simulink model "Receiver_model"  (R2021b)
settings: Solver=FixedStepAuto  StartTime=0  StopTime=70670*4  FixedStep=1  RelTol=1e-3
PostLoadFcn:
  | VarLoad
InitFcn:
  | VarLoad
model workspace: external: MAT-File D:\NIR\WIFI\AGC\Simulink_model\ex1.mat (data not in the file)
undefined symbols (not defined in the file or in its folder): F, magnitude, STF
libraries: simulink x4, dspmathops x1, hdlsllib x1
settings Model: SimulationMode=accelerator  Creator=vadim  LastModifiedBy=vadim

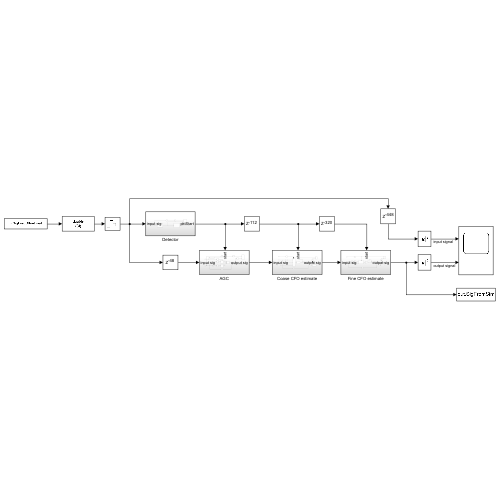
[thumbnail: Simulink's stored preview of the top-level diagram]
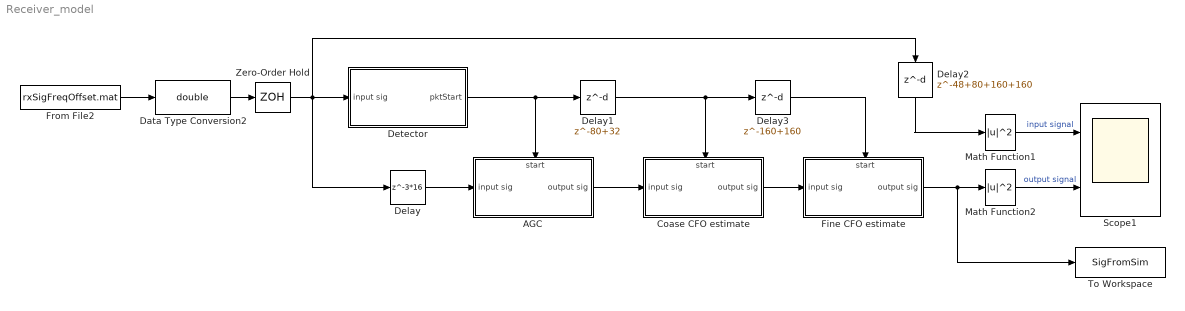
== system Receiver_model ==
  AGC : Subsystem
      settings: PortSchema="{\"entries\":[{\"content\":{\"sides\":[{\"content\":{\"connectorIds\":[\"In1\"]},\"type\":\"ConnectorPlacement.EquallySpacedRectSide\",\"uuid\":\"8c7787f9-30c4-4d5b-a9f2-4534fe769227\"},{\"content\":{\"connectorIds\":[\"Out1\"],\"side\":\"RIGHT\"},\"type\":\"ConnectorPlacement.EquallySpacedRectSide\",\"uuid\":\"2fc322a7-640d-4810-b499-987bf1f99166\"},{\"content\":{\"connectorIds\":[\"In2\"],\"side\":\"TOP\"},\"type\":\"ConnectorPlacement.EquallySpacedRectSide\",\"uuid\":\"709cb384-5402-4f06-933f-6325852d1b42\"}]},\"type\":\"ConnectorPlacement.EquallySpacedConnector\",\"uuid\":\"5f513f7d-d5a1-4295-af52-6e74ab8560d1\"}],\"packageUris\":[\"http://schema.mathworks.com/mf0/Connector/R2020b\"],\"version\":\"1.0\"}"
  Coase CFO estimate : Subsystem
      settings: PortSchema="{\"entries\":[{\"content\":{\"sides\":[{\"content\":{\"connectorIds\":[\"In1\"]},\"type\":\"ConnectorPlacement.EquallySpacedRectSide\",\"uuid\":\"8c7787f9-30c4-4d5b-a9f2-4534fe769227\"},{\"content\":{\"connectorIds\":[\"Out1\"],\"side\":\"RIGHT\"},\"type\":\"ConnectorPlacement.EquallySpacedRectSide\",\"uuid\":\"2fc322a7-640d-4810-b499-987bf1f99166\"},{\"content\":{\"connectorIds\":[\"In2\"],\"side\":\"TOP\"},\"type\":\"ConnectorPlacement.EquallySpacedRectSide\",\"uuid\":\"709cb384-5402-4f06-933f-6325852d1b42\"}]},\"type\":\"ConnectorPlacement.EquallySpacedConnector\",\"uuid\":\"5f513f7d-d5a1-4295-af52-6e74ab8560d1\"}],\"packageUris\":[\"http://schema.mathworks.com/mf0/Connector/R2020b\"],\"version\":\"1.0\"}"
  Data Type Conversion2 : DataTypeConversion  OutDataTypeStr=double  ConvertRealWorld=Stored Integer (SI)
  Delay : Delay  DelayLength=3*16
  Delay1 : Delay  DelayLength=80+32
  Delay2 : Delay  DelayLength=48+80+160+160
  Delay3 : Delay  DelayLength=160+160
  Detector : Subsystem
  Fine CFO estimate : Subsystem
      settings: PortSchema="{\"entries\":[{\"content\":{\"sides\":[{\"content\":{\"connectorIds\":[\"In1\"]},\"type\":\"ConnectorPlacement.EquallySpacedRectSide\",\"uuid\":\"8c7787f9-30c4-4d5b-a9f2-4534fe769227\"},{\"content\":{\"connectorIds\":[\"Out1\"],\"side\":\"RIGHT\"},\"type\":\"ConnectorPlacement.EquallySpacedRectSide\",\"uuid\":\"2fc322a7-640d-4810-b499-987bf1f99166\"},{\"content\":{\"connectorIds\":[\"In2\"],\"side\":\"TOP\"},\"type\":\"ConnectorPlacement.EquallySpacedRectSide\",\"uuid\":\"709cb384-5402-4f06-933f-6325852d1b42\"}]},\"type\":\"ConnectorPlacement.EquallySpacedConnector\",\"uuid\":\"5f513f7d-d5a1-4295-af52-6e74ab8560d1\"}],\"packageUris\":[\"http://schema.mathworks.com/mf0/Connector/R2020b\"],\"version\":\"1.0\"}"
  From File2 : FromFile  FileName=rxSigFreqOffset.mat  SampleTime=0  ExtrapolationAfterLastDataPoint=Ground value
  Math Function1 : Math  Operator=magnitude^2  SaturateOnIntegerOverflow=on
  Math Function2 : Math  Operator=magnitude^2  SaturateOnIntegerOverflow=on
  Scope1 : Scope  NumInputPorts=2
  To Workspace : ToWorkspace  VariableName=SigFromSim  SaveFormat=Timeseries  SampleTime=-1
  Zero-Order Hold : ZeroOrderHold
  wires:
  From File2/1 -> Data Type Conversion2/1
  Data Type Conversion2/1 -> Zero-Order Hold/1
  Delay/1 -> AGC/1(input sig)
  Zero-Order Hold/1 -> Delay/1, Delay2/1, Detector/1(input sig)
  Math Function2/1 -> Scope1/2  "output signal"
  Math Function1/1 -> Scope1/1  "input signal"
  Delay2/1 -> Math Function1/1
  AGC/1(output sig) -> Coase CFO estimate/1(input sig)
  Delay1/1 -> Delay3/1, Coase CFO estimate/2(start)
  Detector/1(pktStart) -> AGC/2(start), Delay1/1
  Coase CFO estimate/1(output sig) -> Fine CFO estimate/1(input sig)
  Fine CFO estimate/1(output sig) -> To Workspace/1, Math Function2/1
  Delay3/1 -> Fine CFO estimate/2(start)

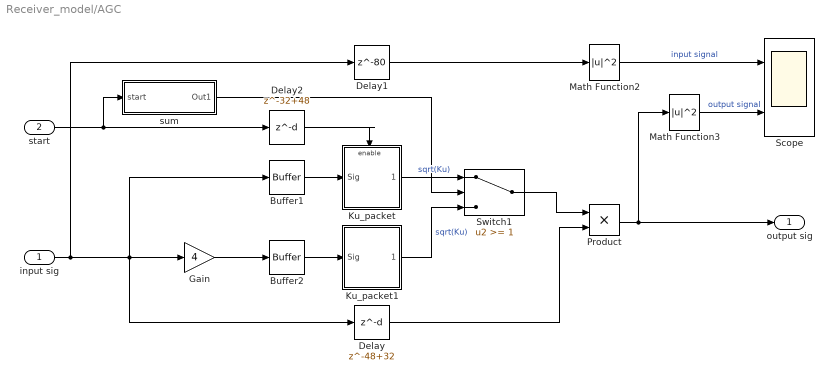
== system Receiver_model/AGC ==
  input sig : Inport
  start : Inport  Port=2
  Buffer1 : Buffer  N=3*16  V=3*16-1  OutputFrames=off
  Buffer2 : Buffer  N=3*16  V=3*16-1  OutputFrames=off
  Delay : Delay  DelayLength=48+32
  Delay1 : Delay  DelayLength=80
  Delay2 : Delay  DelayLength=32+48
  Gain : Gain  Gain=4
  Ku_packet : Subsystem
  Ku_packet1 : Subsystem
  Math Function2 : Math  Operator=magnitude^2  SaturateOnIntegerOverflow=on
  Math Function3 : Math  Operator=magnitude^2  SaturateOnIntegerOverflow=on
  Product : Product
  Scope : Scope  NumInputPorts=2
  Switch1 : Switch  Threshold=1
  sum : Subsystem
  output sig : Outport
  wires:
  Product/1 -> Math Function3/1, output sig/1
  Math Function2/1 -> Scope/1  "input signal"
  Math Function3/1 -> Scope/2  "output signal"
  Ku_packet/1(sqrt(Ku)) -> Switch1/1  "sqrt(Ku)"
  Delay/1 -> Product/2
  Delay1/1 -> Math Function2/1
  Buffer1/1 -> Ku_packet/1(Sig)
  Gain/1 -> Buffer2/1
  input sig/1 -> Delay1/1, Buffer1/1, Delay/1, Gain/1
  Delay2/1 -> Ku_packet/Enable
  Switch1/1 -> Product/1
  Buffer2/1 -> Ku_packet1/1(Sig)
  Ku_packet1/1(sqrt(Ku)) -> Switch1/3  "sqrt(Ku)"
  start/1 -> sum/1(start), Delay2/1
  sum/1(Out1) -> Switch1/2

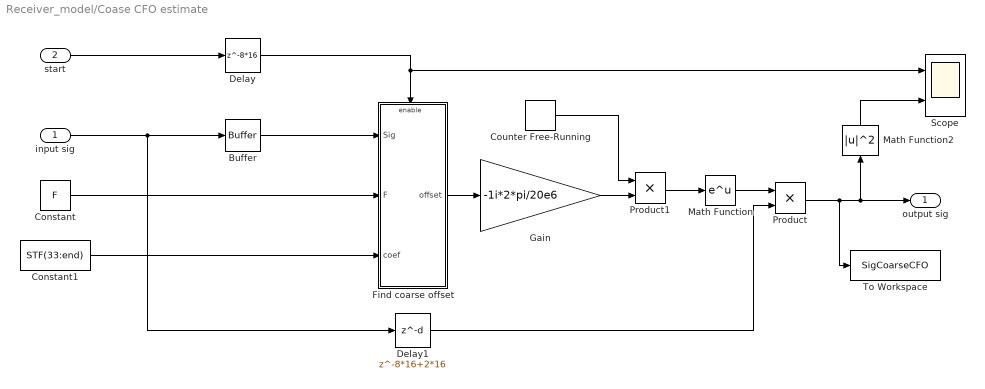
== system Receiver_model/Coase CFO estimate ==
  input sig : Inport
  start : Inport  Port=2
  Buffer : Buffer  N=8*16  V=8*16-1  OutputFrames=off
  Constant : Constant  Value=F
  Constant1 : Constant  Value=STF(33:end)
  Counter Free-Running : simulink/Sources/Counter Free-Running  NumBits=16  tsamp=-1
  Delay : Delay  DelayLength=8*16
  Delay1 : Delay  DelayLength=8*16+2*16
  Find coarse offset : Subsystem
  Gain : Gain  Gain=-1i*2*pi/20e6
  Math Function : Math  SaturateOnIntegerOverflow=on
  Math Function2 : Math  Operator=magnitude^2  SaturateOnIntegerOverflow=on
  Product : Product
  Product1 : Product
  Scope : Scope  NumInputPorts=2
  To Workspace : ToWorkspace  VariableName=SigCoarseCFO  SaveFormat=Timeseries  SampleTime=-1
  output sig : Outport
  wires:
  start/1 -> Delay/1
  input sig/1 -> Buffer/1, Delay1/1
  Gain/1 -> Product1/2
  Math Function/1 -> Product/1
  Delay1/1 -> Product/2
  Product/1 -> To Workspace/1, Math Function2/1, output sig/1
  Delay/1 -> Scope/1, Find coarse offset/Enable
  Buffer/1 -> Find coarse offset/1(Sig)
  Constant/1 -> Find coarse offset/2(F)
  Constant1/1 -> Find coarse offset/3(coef)
  Find coarse offset/1(offset) -> Gain/1
  Math Function2/1 -> Scope/2
  Counter Free-Running/1 -> Product1/1
  Product1/1 -> Math Function/1

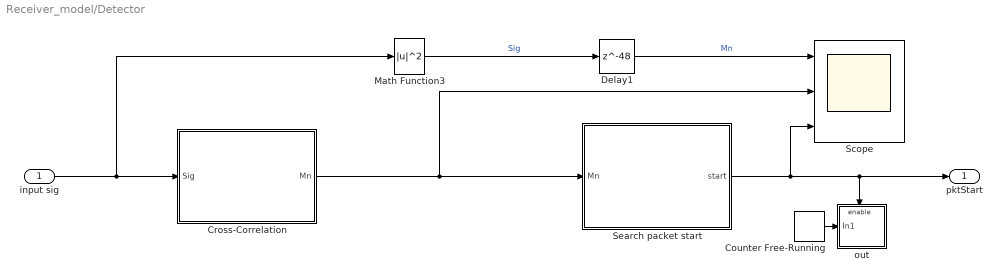
== system Receiver_model/Detector ==
  input sig : Inport
  Counter Free-Running : simulink/Sources/Counter Free-Running  NumBits=32  tsamp=-1
  Cross-Correlation : Subsystem
  Delay1 : Delay  DelayLength=48
  Math Function3 : Math  Operator=magnitude^2  SaturateOnIntegerOverflow=on
  Scope : Scope  NumInputPorts=3
  Search packet start : Subsystem
  out : Subsystem
  pktStart : Outport
  wires:
  Cross-Correlation/1(Mn) -> Scope/2, Search packet start/1(Mn)
  input sig/1 -> Math Function3/1, Cross-Correlation/1(Sig)
  Math Function3/1 -> Delay1/1  "Sig"
  Search packet start/1(start) -> out/Enable, pktStart/1, Scope/3
  Delay1/1 -> Scope/1  "Mn"
  Counter Free-Running/1 -> out/1(In1)

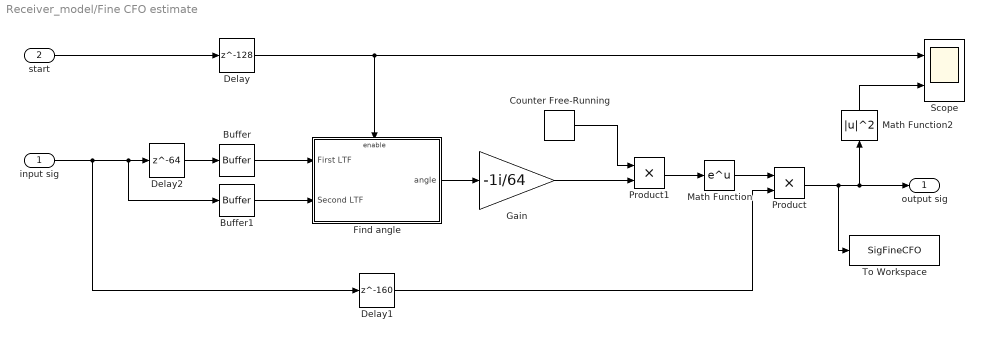
== system Receiver_model/Fine CFO estimate ==
  input sig : Inport
  start : Inport  Port=2
  Buffer : Buffer  V=64-1  OutputFrames=off
  Buffer1 : Buffer  V=64-1  OutputFrames=off
  Counter Free-Running : simulink/Sources/Counter Free-Running  NumBits=16  tsamp=-1
  Delay : Delay  DelayLength=128
  Delay1 : Delay  DelayLength=160
  Delay2 : Delay  DelayLength=64
  Find angle : Subsystem
  Gain : Gain  Gain=-1i/64
  Math Function : Math  SaturateOnIntegerOverflow=on
  Math Function2 : Math  Operator=magnitude^2  SaturateOnIntegerOverflow=on
  Product : Product
  Product1 : Product
  Scope : Scope  NumInputPorts=2
  To Workspace : ToWorkspace  VariableName=SigFineCFO  SaveFormat=Timeseries  SampleTime=-1
  output sig : Outport
  wires:
  start/1 -> Delay/1
  Gain/1 -> Product1/2
  Delay1/1 -> Product/2
  Product/1 -> To Workspace/1, Math Function2/1, output sig/1
  Delay/1 -> Scope/1, Find angle/Enable
  Buffer/1 -> Find angle/1(First LTF)
  Find angle/1(angle) -> Gain/1
  Math Function2/1 -> Scope/2
  Counter Free-Running/1 -> Product1/1
  Product1/1 -> Math Function/1
  Buffer1/1 -> Find angle/2(Second LTF)
  input sig/1 -> Buffer1/1, Delay2/1, Delay1/1
  Delay2/1 -> Buffer/1
  Math Function/1 -> Product/1

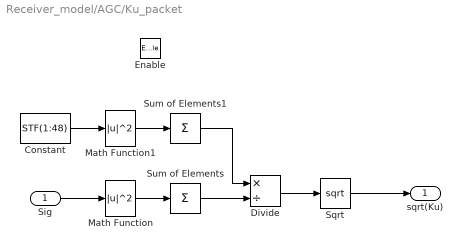
== system Receiver_model/AGC/Ku_packet ==
  Sig : Inport
  Enable : EnablePort
  Constant : Constant  Value=STF(1:48)
  Divide : Product  Inputs=*/
  Math Function : Math  Operator=magnitude^2  SaturateOnIntegerOverflow=on
  Math Function1 : Math  Operator=magnitude^2  SaturateOnIntegerOverflow=on
  Sqrt : Sqrt  SaturateOnIntegerOverflow=on
  Sum of Elements : Sum  Inputs=+
  Sum of Elements1 : Sum  Inputs=+
  sqrt(Ku) : Outport
  wires:
  Sqrt/1 -> sqrt(Ku)/1
  Constant/1 -> Math Function1/1
  Sum of Elements/1 -> Divide/2
  Math Function/1 -> Sum of Elements/1
  Math Function1/1 -> Sum of Elements1/1
  Divide/1 -> Sqrt/1
  Sig/1 -> Math Function/1
  Sum of Elements1/1 -> Divide/1

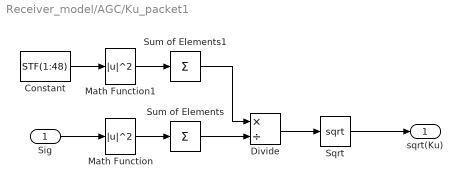
== system Receiver_model/AGC/Ku_packet1 ==
  Sig : Inport
  Constant : Constant  Value=STF(1:48)
  Divide : Product  Inputs=*/
  Math Function : Math  Operator=magnitude^2  SaturateOnIntegerOverflow=on
  Math Function1 : Math  Operator=magnitude^2  SaturateOnIntegerOverflow=on
  Sqrt : Sqrt  SaturateOnIntegerOverflow=on
  Sum of Elements : Sum  Inputs=+
  Sum of Elements1 : Sum  Inputs=+
  sqrt(Ku) : Outport
  wires:
  Sqrt/1 -> sqrt(Ku)/1
  Constant/1 -> Math Function1/1
  Sum of Elements/1 -> Divide/2
  Math Function/1 -> Sum of Elements/1
  Math Function1/1 -> Sum of Elements1/1
  Divide/1 -> Sqrt/1
  Sig/1 -> Math Function/1
  Sum of Elements1/1 -> Divide/1

== system Receiver_model/AGC/sum ==
  start : Inport
  Cumulative Sum : dspmathops/Cumulative Sum  dim=Channels (running sum)  InputProcessing=Columns as channels (frame based)  reset_popup=None  roundingMode=Floor  overflowMode=off  outputDataTypeStr=Inherit: Same as accumulator  outputMin=[]  outputMax=[]  outputLastDataTypeStr=Inherit: Same as accumulator
  Data Type Conversion2 : DataTypeConversion  OutDataTypeStr=double  ConvertRealWorld=Stored Integer (SI)
  Out1 : Outport
  wires:
  Data Type Conversion2/1 -> Cumulative Sum/1
  Cumulative Sum/1 -> Out1/1
  start/1 -> Data Type Conversion2/1

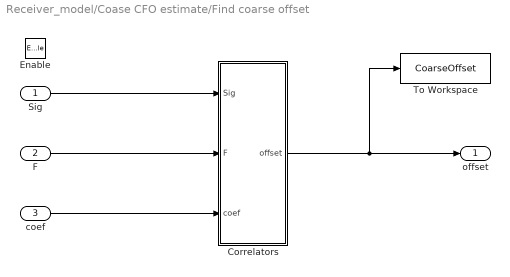
== system Receiver_model/Coase CFO estimate/Find coarse offset ==
  Sig : Inport
  F : Inport  Port=2
  coef : Inport  Port=3
  Enable : EnablePort
  Correlators : MATLAB Function  TreatAsAtomicUnit=on
  To Workspace : ToWorkspace  VariableName=CoarseOffset  SaveFormat=Timeseries  SampleTime=-1
  offset : Outport
  wires:
  Correlators/1(offset) -> To Workspace/1, offset/1
  F/1 -> Correlators/2(F)
  Sig/1 -> Correlators/1(Sig)
  coef/1 -> Correlators/3(coef)

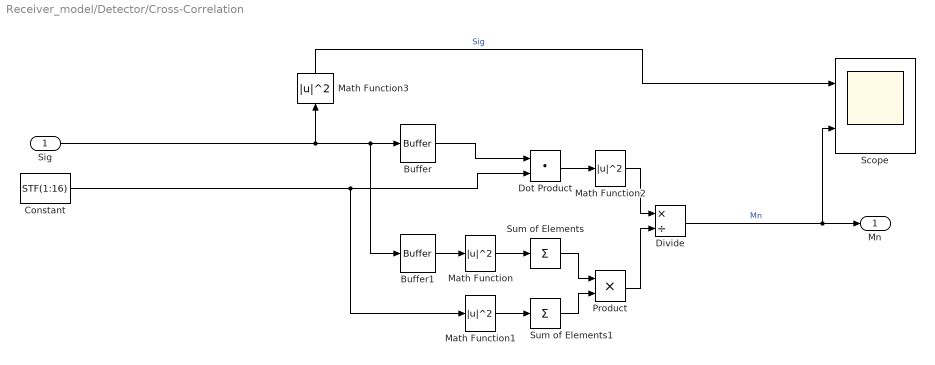
== system Receiver_model/Detector/Cross-Correlation ==
  Sig : Inport
  Buffer : Buffer  N=length(STF(1:16))  V=length(STF(1:16))-1  OutputFrames=off
  Buffer1 : Buffer  N=length(STF(1:16))  V=length(STF(1:16))-1  OutputFrames=off
  Constant : Constant  Value=STF(1:16)
  Divide : Product  Inputs=*/
  Dot Product : DotProduct  InputSameDT=on  OutDataTypeStr=Inherit: Inherit via internal rule
  Math Function{,1..3} (4 alike) : Math  Operator=magnitude^2  SaturateOnIntegerOverflow=on
  Product : Product
  Scope : Scope  NumInputPorts=2
  Sum of Elements : Sum  Inputs=+
  Sum of Elements1 : Sum  Inputs=+
  Mn : Outport
  wires:
  Sig/1 -> Buffer1/1, Buffer/1, Math Function3/1
  Product/1 -> Divide/2
  Dot Product/1 -> Math Function2/1
  Buffer/1 -> Dot Product/1
  Math Function2/1 -> Divide/1
  Divide/1 -> Mn/1, Scope/2  "Mn"
  Buffer1/1 -> Math Function/1
  Constant/1 -> Math Function1/1, Dot Product/2
  Math Function/1 -> Sum of Elements/1
  Math Function1/1 -> Sum of Elements1/1
  Sum of Elements/1 -> Product/1
  Sum of Elements1/1 -> Product/2
  Math Function3/1 -> Scope/1  "Sig"

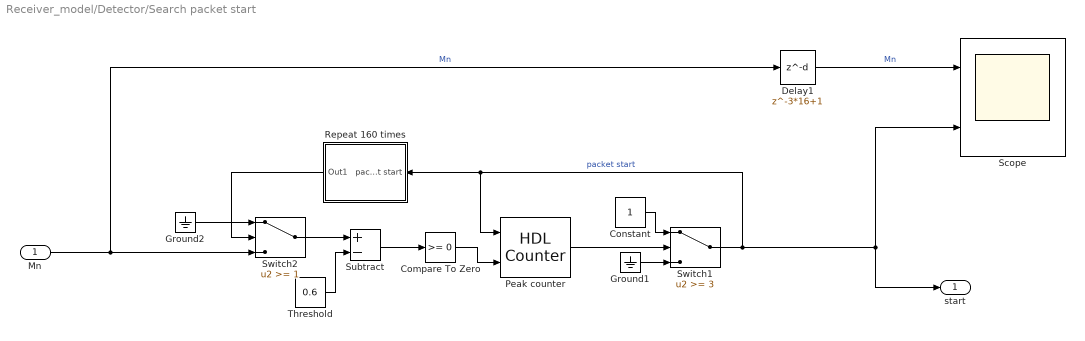
== system Receiver_model/Detector/Search packet start ==
  Mn : Inport
  Compare To Zero : simulink/Logic and Bit Operations/Compare To Zero  relop=>=  OutDataTypeStr=boolean
  Constant : Constant
  Delay1 : Delay  DelayLength=3*16+1
  Ground1 : Ground
  Ground2 : Ground
  Peak counter : hdlsllib/Sources/HDL Counter  CountType=Count limited  CountInit=0  CountStep=1  CountMax=3  CountFromType=Initial value  CountFrom=0  CountResetPort=on  CountLoadPort=off  CountEnbPort=on  CountDirPort=off  CountHitOutputPort=off  CountDataType=Unsigned  CountWordLen=2  CountFracLen=0  CountSampTime=1
  Repeat 160 times : Subsystem
  Scope : Scope  NumInputPorts=2
  Subtract : Sum  Inputs=+-
  Switch1 : Switch  Threshold=3
  Switch2 : Switch  Threshold=1
  Threshold : Constant  Value=0.6
  start : Outport
  wires:
  Threshold/1 -> Subtract/2
  Subtract/1 -> Compare To Zero/1
  Compare To Zero/1 -> Peak counter/2
  Switch1/1 -> start/1, Scope/2, Peak counter/1, Repeat 160 times/1(packet start)  "packet start"
  Ground1/1 -> Switch1/3
  Peak counter/1 -> Switch1/2
  Constant/1 -> Switch1/1
  Mn/1 -> Switch2/3, Delay1/1  "Mn"
  Switch2/1 -> Subtract/1
  Ground2/1 -> Switch2/1
  Delay1/1 -> Scope/1  "Mn"
  Repeat 160 times/1(Out1) -> Switch2/2

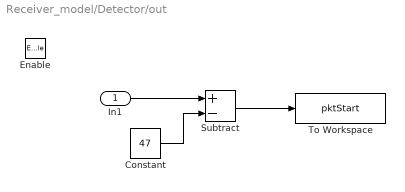
== system Receiver_model/Detector/out ==
  In1 : Inport
  Enable : EnablePort
  Constant : Constant  Value=47
  Subtract : Sum  Inputs=+-
  To Workspace : ToWorkspace  VariableName=pktStart  SaveFormat=Timeseries  SampleTime=-1
  wires:
  In1/1 -> Subtract/1
  Subtract/1 -> To Workspace/1
  Constant/1 -> Subtract/2

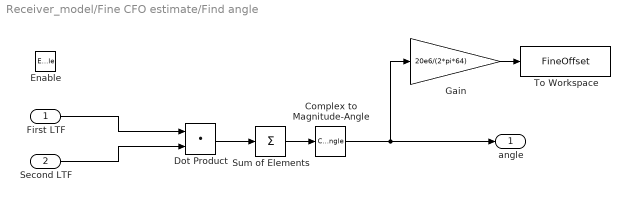
== system Receiver_model/Fine CFO estimate/Find angle ==
  First LTF : Inport
  Second LTF : Inport  Port=2
  Enable : EnablePort
  Complex to Magnitude-Angle : ComplexToMagnitudeAngle  Output=Angle
  Dot Product : DotProduct  InputSameDT=on  OutDataTypeStr=Inherit: Inherit via internal rule
  Gain : Gain  Gain=20e6/(2*pi*64)
  Sum of Elements : Sum  Inputs=+
  To Workspace : ToWorkspace  VariableName=FineOffset  SaveFormat=Timeseries  SampleTime=-1
  angle : Outport
  wires:
  Complex to Magnitude-Angle/1 -> Gain/1, angle/1
  First LTF/1 -> Dot Product/1
  Second LTF/1 -> Dot Product/2
  Dot Product/1 -> Sum of Elements/1
  Sum of Elements/1 -> Complex to Magnitude-Angle/1
  Gain/1 -> To Workspace/1

== system Receiver_model/Detector/Search packet start/Repeat 160 times ==
  packet start : Inport
  Buffer : Buffer  N=160  V=159  OutputFrames=off
  Sum of Elements : Sum  Inputs=+
  Out1 : Outport
  wires:
  packet start/1 -> Buffer/1
  Buffer/1 -> Sum of Elements/1
  Sum of Elements/1 -> Out1/1

== matlab function Receiver_model/Coase CFO estimate/Find coarse offset/Correlators ==
  data: Sig input; F input; coef input; offset output
function offset = fcn(Sig,F,coef)

W = 2*pi*F/20e6;
R = complex(zeros(length(F),1));

for j = 1:length(F)
    coefWithOffset = coef.*exp(1i*W(j)*(33:160)');
    R(j) = sum(conj(Sig).*coefWithOffset);
end

[~,ind] = max(R);
offset = F(ind);
